simulink library "Lib_Cntrl_GainSchedulerD2D_TMATS"  (R2019b)
settings: Solver=ode45  StartTime=0.0  StopTime=10.0  RelTol=1e-3  EnableMultiTasking=on
Description:
  | Thomas Modules
settings Model: Creator=jwchapm2  LastModifiedBy=bhisma
settings DataIOCC: LimitDataPoints=on  SaveFormat=Array  ReturnWorkspaceOutputs=off
settings OptimizationCC: ExpressionDepthLimit=2147483647  LifeSpan=inf
settings DebuggingCC: UnderspecifiedInitializationDetection=Classic  MergeDetectMultiDrivingBlocksExec=none  SolverPrmCheckMsg=warning  StateNameClashWarn=warning  SFUnexpectedBacktrackingDiag=warning  SFNoUnconditionalDefaultTransitionDiag=warning  SFExecutionAtInitializationDiag=none  ArithmeticOperatorsInVariantConditions=warning
settings HardwareCC: ProdBitPerPointer=32  ProdBitPerSizeT=32  ProdBitPerPtrDiffT=32  ProdLargestAtomicFloat=None  ProdIntDivRoundTo=Undefined  ProdEndianess=Unspecified  ProdWordSize=32  ProdHWDeviceType=32-bit Generic
settings ModelReferenceCC: PropagateSignalLabelsOutOfModel=off
settings SFSimCC: SimUseLocalCustomCode=off  CustomCodeUndefinedFunction=UseInterfaceOnly
settings RTWCC: RTWUseLocalCustomCode=off
settings CodeAppCC: StateflowObjectComments=on
settings GRTTargetCC: TargetLangStandard=C89/C90 (ANSI)  GeneratePreprocessorConditionals=Disable all
settings ConfigComp: CovMetricSettings=dw  CovHtmlReporting=on  CovSaveCumulativeToWorkspaceVar=on  CovSaveSingleToWorkspaceVar=on  CovExternalEMLEnable=off

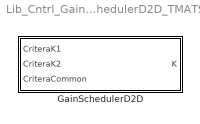
== system Lib_Cntrl_GainSchedulerD2D_TMATS ==
  GainSchedulerD2D : Subsystem  mask(T-MATS: Gain Scheduler D2D){CCVec_M=[1 2], CK1Vec_M=[1 2 3], K1Array_M=[1 1; 1 1; 1 1], CK2Vec_M=[1 2 3 4], K2Array_M=[1 1; 1 1; 1 1; 1 1]}
      mask prompts: CCVec_M "CCVec_M - Common Critera Vector (1xn)"; CK1Vec_M "CK1Vec_M - Critera for gain 1 (1xm)"; K1Array_M "K1Array_M - Gain 1 array (mxn)"; CK2Vec_M "CK2Vec_M - Critera for gain 2 (1xp)"; K2Array_M "K2Array_M_M - Gain 2 array (pxn)"
      mask help: This block a double 2 dimensional gain scheduler. Input are two critera and a common critera that are used for two 2-D lookups. Output contains the result of the table lookups. In general these two results will be multiplied together and can be entered into either the Ki or Kp input of the T-MATS setpoint controller block. Additionally the outputs could be separated and used as inputs to both Kp and Ki.
      mask Help: web(which('Control_TMATS_GSD2D.html'),'-helpbrowser')

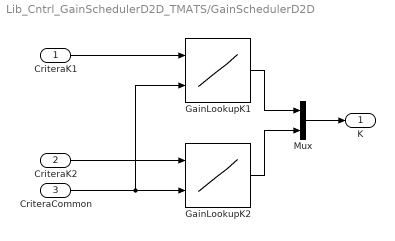
== system Lib_Cntrl_GainSchedulerD2D_TMATS/GainSchedulerD2D ==
  CriteraK1 : Inport
  CriteraK2 : Inport  Port=2
  CriteraCommon : Inport  Port=3
  GainLookupK1 : Lookup_n-D  BreakpointsForDimension1=CK1Vec_M  BreakpointsForDimension2=CCVec_M  Table=K1Array_M  InterpMethod=Nearest  DiagnosticForOutOfRangeInput=Warning  InternalRulePriority=Speed  RndMeth=Simplest  InputSameDT=on
  GainLookupK2 : Lookup_n-D  BreakpointsForDimension1=CK2Vec_M  BreakpointsForDimension2=CCVec_M  Table=K2Array_M  InterpMethod=Flat  DiagnosticForOutOfRangeInput=Warning  InternalRulePriority=Speed  RndMeth=Simplest  InputSameDT=on
  Mux : Mux  Inputs=2
  K : Outport
  wires:
  CriteraCommon/1 -> GainLookupK1/2, GainLookupK2/2
  CriteraK1/1 -> GainLookupK1/1
  Mux/1 -> K/1
  CriteraK2/1 -> GainLookupK2/1
  GainLookupK1/1 -> Mux/1
  GainLookupK2/1 -> Mux/2
